simulink model "lin_model_3"  (R2022b)
settings: Solver=VariableStepAuto  StartTime=0.0  StopTime=10  RelTol=1e-3
values from neighbouring files (symbols this model uses):
  A = double(A)    [dyn_model_mark.m]
  B = double(B)    [dyn_model_mark.m]
  C = [1 0 0 0 ... (first row only)    [dyn_model_mark.m]
  D = [0 ... (first row only)    [dyn_model_mark.m]
  Va_bar = double(sol)    [dyn_model_mark.m]
  x1_bar = 0    [dyn_model_mark.m]
  x3_bar = pi    (= 3.14159265359)    [dyn_model_mark.m]
settings Model: Creator=Mark  LastModifiedBy=Mark
settings OptimizationCC: ReuseModelBlockBuffer=on

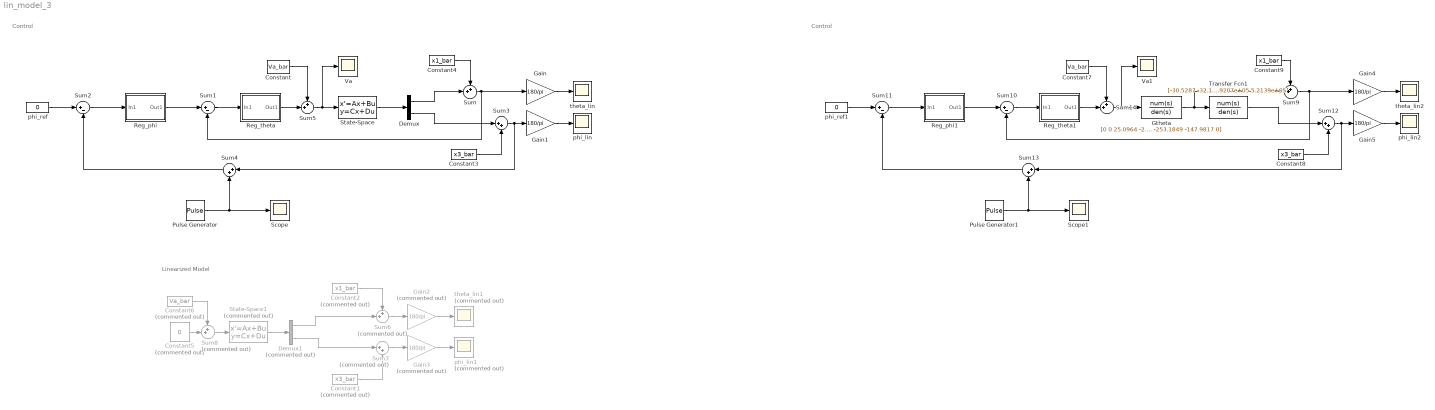
== system lin_model_3 ==
  note: Control
  note: Linearized Model
  note: Control
  Constant : Constant  Value=Va_bar
  Constant1 : Constant  Commented=on  Value=x3_bar
  Constant2 : Constant  Commented=on  Value=x1_bar
  Constant3 : Constant  Value=x3_bar
  Constant4 : Constant  Value=x1_bar
  Constant5 : Constant  Commented=on  Value=0
  Constant6 : Constant  Commented=on  Value=Va_bar
  Constant7 : Constant  Value=Va_bar
  Constant8 : Constant  Value=x3_bar
  Constant9 : Constant  Value=x1_bar
  Demux : Demux  Outputs=2
  Demux1 : Demux  Commented=on  Outputs=2
  Gain{,1,4..5} (4 alike) : Gain  Gain=180/pi
  Gain2 : Gain  Commented=on  Gain=180/pi
  Gain3 : Gain  Commented=on  Gain=180/pi
  Gtheta : TransferFcn  Numerator=[0 0 25.0964 -2.6748e-13 -3.5234e+03]  Denominator=[1 1.0540 -253.1849 -147.9817 0]
  Pulse Generator : DiscretePulseGenerator  PulseType=Time based  Period=10000  PulseWidth=0.01  PhaseDelay=1
  Pulse Generator1 : DiscretePulseGenerator  PulseType=Time based  Period=10000  PulseWidth=0.01  PhaseDelay=1
  Reg_phi : Subsystem
  Reg_phi1 : Subsystem
  Reg_theta : Subsystem
  Reg_theta1 : Subsystem
  Scope : Scope
  Scope1 : Scope
  State-Space : StateSpace  A=A  B=B  C=C  D=D  InitialCondition=[0 0 0 0]  ParameterTunability=Optimized
  State-Space1 : StateSpace  Commented=on  A=A  B=B  C=C  D=D  InitialCondition=[0 0 pi/2 0]  ParameterTunability=Optimized
  Sum{,5,9,14} (4 alike) : Sum  Inputs=++|
  Sum{1..2,10..11} (4 alike) : Sum  Inputs=|+-
  Sum{3..4,12..13} (4 alike) : Sum  Inputs=|++
  Sum6 : Sum  Commented=on  Inputs=++|
  Sum7 : Sum  Commented=on  Inputs=|++
  Sum8 : Sum  Commented=on  Inputs=++|
  Transfer Fcn1 : TransferFcn  Numerator=[-30.5287 -32.1788 7.7294e+03 4.5177e+03 2.6254e-12 0]  Denominator=[25.0964 26.4528 -9.8774e+03 -7.4276e+03 8.9207e+05 5.2139e+05]
  Va : Scope
  Va1 : Scope
  phi_lin : Scope
  phi_lin1 : Scope  Commented=on
  phi_lin2 : Scope
  phi_ref : Constant  Value=0
  phi_ref1 : Constant  Value=0
  theta_lin : Scope
  theta_lin1 : Scope  Commented=on
  theta_lin2 : Scope
  wires:
  phi_ref/1 -> Sum2/1
  Reg_phi/1(Out1) -> Sum1/1
  Sum2/1 -> Reg_phi/1(In1)
  State-Space/1 -> Demux/1
  Gain/1 -> theta_lin/1
  Gain1/1 -> phi_lin/1
  Sum/1 -> Gain/1, Sum1/2
  Sum3/1 -> Sum4/1, Gain1/1
  Constant3/1 -> Sum3/2
  Constant4/1 -> Sum/1
  Demux/1 -> Sum/2
  Demux/2 -> Sum3/1
  Sum5/1 -> Va/1, State-Space/1
  Sum1/1 -> Reg_theta/1(In1)
  Sum4/1 -> Sum2/2
  Pulse Generator/1 -> Scope/1, Sum4/2
  Reg_theta/1(Out1) -> Sum5/2
  Constant/1 -> Sum5/1
  Demux1/2 -> Sum7/1
  Sum7/1 -> Gain3/1
  Gain3/1 -> phi_lin1/1
  State-Space1/1 -> Demux1/1
  Demux1/1 -> Sum6/2
  Constant2/1 -> Sum6/1
  Gain2/1 -> theta_lin1/1
  Constant1/1 -> Sum7/2
  Sum6/1 -> Gain2/1
  Constant5/1 -> Sum8/2
  Sum8/1 -> State-Space1/1
  Constant6/1 -> Sum8/1
  phi_ref1/1 -> Sum11/1
  Sum13/1 -> Sum11/2
  Gain5/1 -> phi_lin2/1
  Sum10/1 -> Reg_theta1/1(In1)
  Constant9/1 -> Sum9/1
  Sum9/1 -> Gain4/1, Sum10/2
  Sum14/1 -> Gtheta/1, Va1/1
  Reg_theta1/1(Out1) -> Sum14/2
  Pulse Generator1/1 -> Scope1/1, Sum13/2
  Gain4/1 -> theta_lin2/1
  Sum11/1 -> Reg_phi1/1(In1)
  Reg_phi1/1(Out1) -> Sum10/1
  Sum12/1 -> Sum13/1, Gain5/1
  Constant8/1 -> Sum12/2
  Constant7/1 -> Sum14/1
  Gtheta/1 -> Sum9/2, Transfer Fcn1/1
  Transfer Fcn1/1 -> Sum12/1

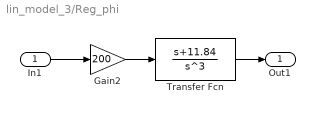
== system lin_model_3/Reg_phi ==
  In1 : Inport
  Gain2 : Gain  Gain=200
  Transfer Fcn : TransferFcn  Numerator=[1 11.84]  Denominator=[1 0 0 0]
  Out1 : Outport
  wires:
  Gain2/1 -> Transfer Fcn/1
  Transfer Fcn/1 -> Out1/1
  In1/1 -> Gain2/1

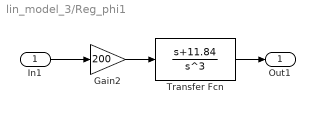
== system lin_model_3/Reg_phi1 ==
  In1 : Inport
  Gain2 : Gain  Gain=200
  Transfer Fcn : TransferFcn  Numerator=[1 11.84]  Denominator=[1 0 0 0]
  Out1 : Outport
  wires:
  Gain2/1 -> Transfer Fcn/1
  Transfer Fcn/1 -> Out1/1
  In1/1 -> Gain2/1

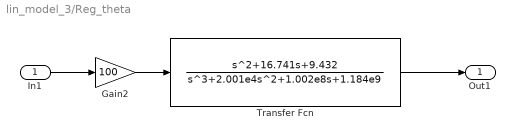
== system lin_model_3/Reg_theta ==
  In1 : Inport
  Gain2 : Gain  Gain=100
  Transfer Fcn : TransferFcn  Numerator=[1 16.741 9.432]  Denominator=[1 2.001e4 1.002e8 1.184e9]
  Out1 : Outport
  wires:
  Gain2/1 -> Transfer Fcn/1
  Transfer Fcn/1 -> Out1/1
  In1/1 -> Gain2/1

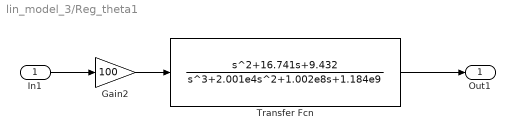
== system lin_model_3/Reg_theta1 ==
  In1 : Inport
  Gain2 : Gain  Gain=100
  Transfer Fcn : TransferFcn  Numerator=[1 16.741 9.432]  Denominator=[1 2.001e4 1.002e8 1.184e9]
  Out1 : Outport
  wires:
  Gain2/1 -> Transfer Fcn/1
  Transfer Fcn/1 -> Out1/1
  In1/1 -> Gain2/1
